simulink model "Expt_1_a"  (R2018a)
settings: Solver=VariableStepAuto  StartTime=0.0  StopTime=10.0  RelTol=1e-3
settings Model: Creator=HP  LastModifiedBy=HP

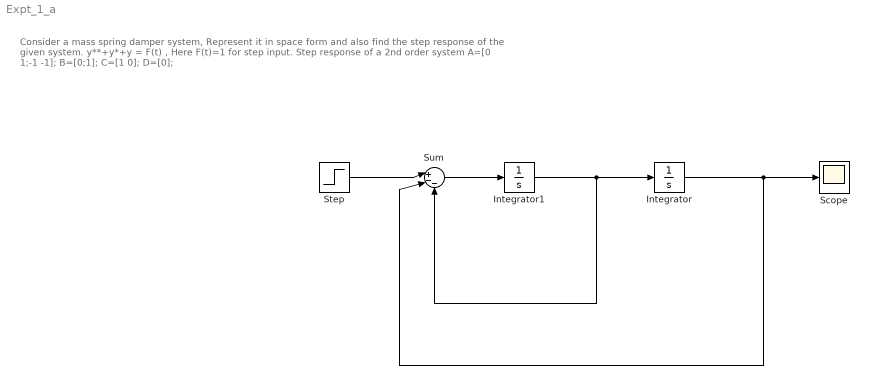
== system Expt_1_a ==
  note: Consider a mass spring damper system, Represent it in space form and also
      | find the step response of the given system.
      | y**+y*+y = F(t) , Here F(t)=1 for step input.
      |
      | Step response of a 2nd order system
      |
      | A=[0 1;-1 -1];
      | B=[0;1];
      | C=[1 0];
      | D=[0];
  Integrator : Integrator
  Integrator1 : Integrator
  Scope : Scope
  Step : Step  SampleTime=0
  Sum : Sum  Inputs=|+--
  wires:
  Step/1 -> Sum/1
  Sum/1 -> Integrator1/1
  Integrator/1 -> Scope/1, Sum/2
  Integrator1/1 -> Sum/3, Integrator/1
